simulink model "IMU_nav"  (Simulink 8.0)
settings: Solver=ode45  StartTime=0.0  StopTime=10.0  RelTol=1e-3
values from neighbouring files (symbols this model uses):
  TSample = T_sim    [IMU_param.m]
undefined symbols (not defined in the file or in its folder): ACCEL, GYRO
settings Model: Creator=Victor  LastModifiedBy=David
settings DataIOCC: SignalLoggingSaveFormat=ModelDataLogs
settings DebuggingCC: FcnCallInpInsideContextMsg=UseLocalSettings
settings GRTTargetCC: CombineOutputUpdateFcns=off  GRTInterface=on

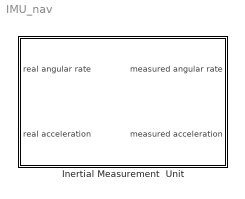
== system IMU_nav ==
  Inertial Measurement  Unit : Subsystem

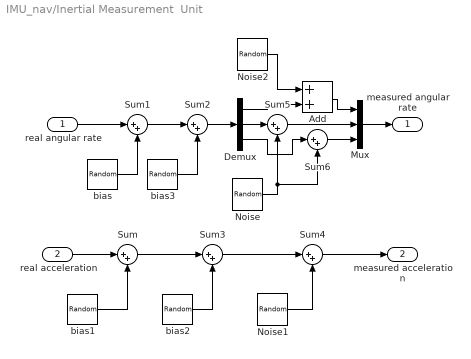
== system IMU_nav/Inertial Measurement  Unit ==
  real angular rate : Inport
  real acceleration : Inport  Port=2
  Add : Sum
  Demux : Demux  Outputs=3
  Mux : Mux  Inputs=3
  Noise : UniformRandomNumber  Minimum=-GYRO.noise_pith  Maximum=GYRO.noise_pith  Seed=346  SampleTime=TSample
  Noise1 : UniformRandomNumber  Minimum=-ACCEL.noise  Maximum=ACCEL.noise  Seed=134  SampleTime=TSample
  Noise2 : UniformRandomNumber  Minimum=-GYRO.noise_roll  Maximum=GYRO.noise_roll  Seed=98  SampleTime=TSample
  Sum{,1..6} (7 alike) : Sum  Inputs=|++
  bias : RandomNumber  Variance=GYRO.bias_repeat  Seed=245  SampleTime=TSample
  bias1 : RandomNumber  Variance=ACCEL.bias_repeat  Seed=43  SampleTime=TSample
  bias2 : RandomNumber  Variance=ACCEL.bias_stability  Seed=472  SampleTime=TSample
  bias3 : RandomNumber  Variance=GYRO.bias_stability  Seed=734  SampleTime=TSample
  measured angular rate : Outport
  measured acceleration : Outport  Port=2
  wires:
  real acceleration/1 -> Sum/1
  real angular rate/1 -> Sum1/1
  Sum1/1 -> Sum2/1
  Mux/1 -> measured angular rate/1
  Sum/1 -> Sum3/1
  Sum3/1 -> Sum4/1
  Sum4/1 -> measured acceleration/1
  bias1/1 -> Sum/2
  bias2/1 -> Sum3/2
  Noise1/1 -> Sum4/2
  Sum2/1 -> Demux/1
  bias3/1 -> Sum2/2
  bias/1 -> Sum1/2
  Demux/2 -> Sum5/1
  Noise/1 -> Sum5/2, Sum6/2
  Demux/3 -> Sum6/1
  Sum6/1 -> Mux/3
  Sum5/1 -> Mux/2
  Noise2/1 -> Add/1
  Demux/1 -> Add/2
  Add/1 -> Mux/1
